simulink model "AWD_EV_MODEL_rev2_SMC"  (Simulink 8.7)
settings: Solver=ode3  SolverMode=SingleTasking  StartTime=0.0  StopTime=20  FixedStep=0.001  RelTol=1e-3
undefined symbols (not defined in the file): Bx, Bx_2, By, By_2, Cx, Cx_2, Cy, Cy_2, Dx, Dx_2, Dy, Dy_2, Ex, Ex_2, Ey, Ey_2, g, GRR, GRR_E, hg, Ixx, Iyy, Jw, Jz, Lf, Lr, Lw, m, r0, Rw, rx1, rx1_2, rx2, rx2_2, ry1, ry1_2, ry2, ry2_2, SA_A, SA_SAT_n, SA_SAT_p, SA_Slope, sigbuilder_block, Split_u_Time_On, SR_Eq_Accel_Brake_Threshold, Steering_Input_Select, T_Avail, Throttle_Final_Val, Throttle_Init_Val, Throttle_Step_Time, Vx0, Vy0, wRL0, z
libraries: simulink x10
(part 2 of 2)

== system AWD_EV_MODEL_rev2_SMC/FL Tire Mode/Magic Formula/Magic Formula Condition 1 ==
  Slip ratio : Inport
  Slip angle [rad] : Inport  Port=2
  Bgx : Fcn  Expr=rx1*cos(atan(rx2*u))
  Bgy : Fcn  Expr=ry1*cos(atan(ry2*u))
  Gx : Fcn  Expr=cos(atan(u))
  Gy : Fcn  Expr=cos(atan(u))
  Product{,1..3} (4 alike) : Product  RndMeth=Zero
  u-a curve : Fcn  Expr=Dy*sin(Cy*atan(By*u-Ey*(By*u-atan(By*u))))
  u-a curve4 : Fcn  Expr=tan(u)
  u-s curve : Fcn  Expr=Dx*sin(Cx*atan(Bx*u-Ex*(Bx*u-atan(Bx*u))))
  Long. friction coefficient : Outport
  Lat. friction coefficient : Outport  Port=2
  wires:
  Bgx/1 -> Product/2
  Bgy/1 -> Product2/2
  Slip angle [rad]/1 -> u-a curve4/1
  Product3/1 -> Lat. friction coefficient/1  "combined"
  Gy/1 -> Product3/1
  Product2/1 -> Gy/1
  Product1/1 -> Long. friction coefficient/1  "combined"
  Gx/1 -> Product1/2
  Product/1 -> Gx/1
  u-a curve4/1 -> Product/1, Bgy/1, u-a curve/1
  Slip ratio/1 -> Bgx/1, Product2/1, u-s curve/1
  u-a curve/1 -> Product3/2  "Muy"
  u-s curve/1 -> Product1/1  "Mux"

== system AWD_EV_MODEL_rev2_SMC/FL Tire Mode/Magic Formula/Magic Formula Condition 2 ==
  Slip ratio : Inport
  Slip angle [rad] : Inport  Port=2
  Bgx : Fcn  Expr=rx1_2*cos(atan(rx2_2*u))
  Bgy : Fcn  Expr=ry1_2*cos(atan(ry2_2*u))
  Gx : Fcn  Expr=cos(atan(u))
  Gy : Fcn  Expr=cos(atan(u))
  Product{,1..3} (4 alike) : Product  RndMeth=Zero
  u-a curve : Fcn  Expr=Dy_2*sin(Cy_2*atan(By_2*u-Ey_2*(By_2*u-atan(By_2*u))))
  u-a curve4 : Fcn  Expr=tan(u)
  u-s curve : Fcn  Expr=Dx_2*sin(Cx_2*atan(Bx_2*u-Ex_2*(Bx_2*u-atan(Bx_2*u))))
  Long. friction coefficient : Outport
  Lat. friction coefficient : Outport  Port=2
  wires:
  Bgx/1 -> Product/2
  Bgy/1 -> Product2/2
  Slip angle [rad]/1 -> u-a curve4/1
  Product3/1 -> Lat. friction coefficient/1  "combined"
  Gy/1 -> Product3/1
  Product2/1 -> Gy/1
  Product1/1 -> Long. friction coefficient/1  "combined"
  Gx/1 -> Product1/2
  Product/1 -> Gx/1
  u-a curve4/1 -> Product/1, Bgy/1, u-a curve/1
  Slip ratio/1 -> Bgx/1, Product2/1, u-s curve/1
  u-a curve/1 -> Product3/2  "Muy"
  u-s curve/1 -> Product1/1  "Mux"

== system AWD_EV_MODEL_rev2_SMC/FR Tire Mode/Magic Formula1/Magic Formula Condition 1 ==
  Slip ratio : Inport
  Slip angle [rad] : Inport  Port=2
  Bgx : Fcn  Expr=rx1*cos(atan(rx2*u))
  Bgy : Fcn  Expr=ry1*cos(atan(ry2*u))
  Gx : Fcn  Expr=cos(atan(u))
  Gy : Fcn  Expr=cos(atan(u))
  Product{,1..3} (4 alike) : Product  RndMeth=Zero
  u-a curve : Fcn  Expr=Dy*sin(Cy*atan(By*u-Ey*(By*u-atan(By*u))))
  u-a curve4 : Fcn  Expr=tan(u)
  u-s curve : Fcn  Expr=Dx*sin(Cx*atan(Bx*u-Ex*(Bx*u-atan(Bx*u))))
  Long. friction coefficient : Outport
  Lat. friction coefficient : Outport  Port=2
  wires:
  Bgx/1 -> Product/2
  Bgy/1 -> Product2/2
  Slip angle [rad]/1 -> u-a curve4/1
  Product3/1 -> Lat. friction coefficient/1  "combined"
  Gy/1 -> Product3/1
  Product2/1 -> Gy/1
  Product1/1 -> Long. friction coefficient/1  "combined"
  Gx/1 -> Product1/2
  Product/1 -> Gx/1
  u-a curve4/1 -> Product/1, Bgy/1, u-a curve/1
  Slip ratio/1 -> Bgx/1, Product2/1, u-s curve/1
  u-a curve/1 -> Product3/2  "Muy"
  u-s curve/1 -> Product1/1  "Mux"

== system AWD_EV_MODEL_rev2_SMC/FR Tire Mode/Magic Formula1/Magic Formula Condition 2 ==
  Slip ratio : Inport
  Slip angle [rad] : Inport  Port=2
  Bgx : Fcn  Expr=rx1_2*cos(atan(rx2_2*u))
  Bgy : Fcn  Expr=ry1_2*cos(atan(ry2_2*u))
  Gx : Fcn  Expr=cos(atan(u))
  Gy : Fcn  Expr=cos(atan(u))
  Product{,1..3} (4 alike) : Product  RndMeth=Zero
  u-a curve : Fcn  Expr=Dy_2*sin(Cy_2*atan(By_2*u-Ey_2*(By_2*u-atan(By_2*u))))
  u-a curve4 : Fcn  Expr=tan(u)
  u-s curve : Fcn  Expr=Dx_2*sin(Cx_2*atan(Bx_2*u-Ex_2*(Bx_2*u-atan(Bx_2*u))))
  Long. friction coefficient : Outport
  Lat. friction coefficient : Outport  Port=2
  wires:
  Bgx/1 -> Product/2
  Bgy/1 -> Product2/2
  Slip angle [rad]/1 -> u-a curve4/1
  Product3/1 -> Lat. friction coefficient/1  "combined"
  Gy/1 -> Product3/1
  Product2/1 -> Gy/1
  Product1/1 -> Long. friction coefficient/1  "combined"
  Gx/1 -> Product1/2
  Product/1 -> Gx/1
  u-a curve4/1 -> Product/1, Bgy/1, u-a curve/1
  Slip ratio/1 -> Bgx/1, Product2/1, u-s curve/1
  u-a curve/1 -> Product3/2  "Muy"
  u-s curve/1 -> Product1/1  "Mux"

== system AWD_EV_MODEL_rev2_SMC/Wheel States1/Subsystem1/negative slip angle ==
  in : Inport
  Action Port : ActionPort  ActionType=else
  Gain : Gain  Gain=-1
  -in : Outport
  wires:
  in/1 -> Gain/1
  Gain/1 -> -in/1

== system AWD_EV_MODEL_rev2_SMC/Wheel States1/Subsystem1/positive slip angle ==
  in : Inport
  Action Port : ActionPort  ActionType=then
  +in : Outport
  wires:
  in/1 -> +in/1

== system AWD_EV_MODEL_rev2_SMC/Wheel States1/Subsystem2/negative slip angle ==
  in : Inport
  Action Port : ActionPort  ActionType=else
  Gain : Gain  Gain=-1
  -in : Outport
  wires:
  Gain/1 -> -in/1
  in/1 -> Gain/1

== system AWD_EV_MODEL_rev2_SMC/Wheel States1/Subsystem2/positive slip angle ==
  in : Inport
  Action Port : ActionPort  ActionType=then
  +in : Outport
  wires:
  in/1 -> +in/1

== system AWD_EV_MODEL_rev2_SMC/Wheel States1/Subsystem3/negative slip angle ==
  in : Inport
  Action Port : ActionPort  ActionType=else
  Gain : Gain  Gain=-1
  -in : Outport
  wires:
  Gain/1 -> -in/1
  in/1 -> Gain/1

== system AWD_EV_MODEL_rev2_SMC/Wheel States1/Subsystem3/positive slip angle ==
  in : Inport
  Action Port : ActionPort  ActionType=then
  +in : Outport
  wires:
  in/1 -> +in/1

== system AWD_EV_MODEL_rev2_SMC/Wheel States1/Subsystem4/negative slip angle ==
  in : Inport
  Action Port : ActionPort  ActionType=else
  Gain : Gain  Gain=-1
  -in : Outport
  wires:
  in/1 -> Gain/1
  Gain/1 -> -in/1

== system AWD_EV_MODEL_rev2_SMC/Wheel States1/Subsystem4/positive slip angle ==
  in : Inport
  Action Port : ActionPort  ActionType=then
  +in : Outport
  wires:
  in/1 -> +in/1

== matlab function MATLAB Function1 ==
  data: u input double
function fcn(u)
%#codegen
rectangle('Position',[5 -1 2 2]);
rectangle('Position',[5 29 2 2]);
rectangle('Position',[5 59 2 2]);
rectangle('Position',[5 89 2 2]);
rectangle('Position',[5 119 2 2]);
rectangle('Position',[5 149 2 2]);
rectangle('Position',[5 179 2 2]);

== matlab function MATLAB Function ==
  data: x input double; y input double
function fcn(x,y)
%#codegen
%coder.extrinsic('rectangle')
%rectangle('Position',[1 2 5 6]);
%rectangle('Position',[10 2 5 6]);
%coder.extrinsic('plot')
plot(x,y,'s','Markersize',8,'MarkerFaceColor','g');
%plot(x,y,'s','Markersize',8,'MarkerFaceColor','g','erasemode','background')
%plot(x,y)
set(gca,'XLim',[-50+x 50+x],'Ylim',[-20+y 100+y]) % or whatever axes limits you want
grid on
